simulink model "prob2"  (R2020b)
settings: Solver=VariableStepAuto  StartTime=0.0  StopTime=10.0  RelTol=1e-3
undefined symbols (not defined in the file): b, k1, k2, M1, M2
settings Model: Creator=nadee  LastModifiedBy=nadee

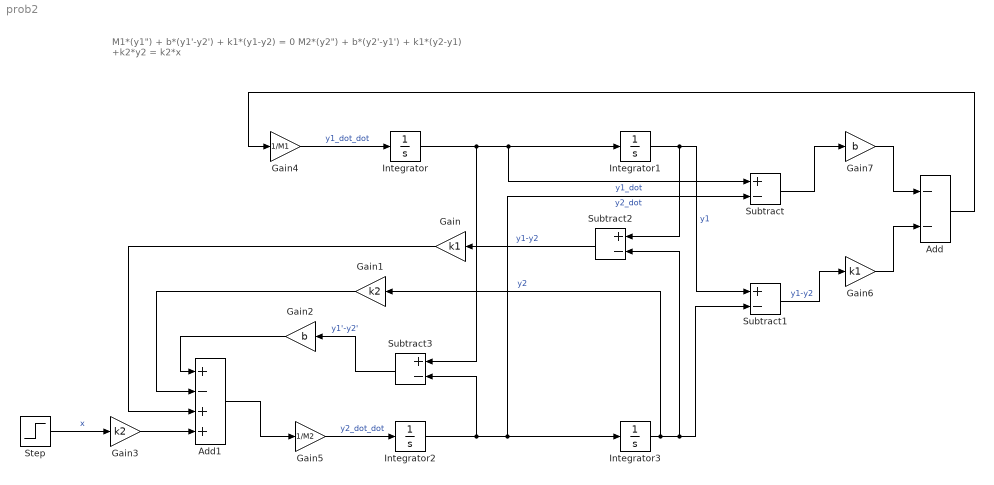
== system prob2 ==
  note: M1*(y1") + b*(y1'-y2') + k1*(y1-y2) = 0
      | M2*(y2") + b*(y2'-y1') + k1*(y2-y1) +k2*y2 = k2*x
  Add : Sum  Inputs=--
  Add1 : Sum  Inputs=+-++
  Gain : Gain  Gain=k1
  Gain1 : Gain  Gain=k2
  Gain2 : Gain  Gain=b
  Gain3 : Gain  Gain=k2
  Gain4 : Gain  Gain=1/M1
  Gain5 : Gain  Gain=1/M2
  Gain6 : Gain  Gain=k1
  Gain7 : Gain  Gain=b
  Integrator{,1..3} (4 alike) : Integrator
  Step : Step  SampleTime=0
  Subtract{,1..3} (4 alike) : Sum  Inputs=+-
  wires:
  Gain4/1 -> Integrator/1  "y1_dot_dot"
  Integrator/1 -> Subtract3/1, Subtract/1, Integrator1/1  "y1_dot"
  Integrator1/1 -> Subtract2/1, Subtract1/1  "y1"
  Integrator3/1 -> Gain1/1, Subtract2/2, Subtract1/2  "y2"
  Integrator2/1 -> Subtract/2, Integrator3/1, Subtract3/2  "y2_dot"
  Gain5/1 -> Integrator2/1  "y2_dot_dot"
  Add1/1 -> Gain5/1
  Subtract1/1 -> Gain6/1  "y1-y2"
  Gain6/1 -> Add/2
  Subtract/1 -> Gain7/1
  Gain7/1 -> Add/1
  Add/1 -> Gain4/1
  Subtract2/1 -> Gain/1  "y1-y2"
  Gain/1 -> Add1/3
  Gain1/1 -> Add1/2
  Gain2/1 -> Add1/1
  Subtract3/1 -> Gain2/1  "y1'-y2'"
  Step/1 -> Gain3/1  "x"
  Gain3/1 -> Add1/4
